simulink model "Modello1DoF_alessio"  (R2023a)
settings: Solver=ode1  StartTime=0.0  StopTime=20  FixedStep=0.001  RelTol=1e-3
libraries: autolibshared x1
settings Model: Creator=salvo  LastModifiedBy=alessio

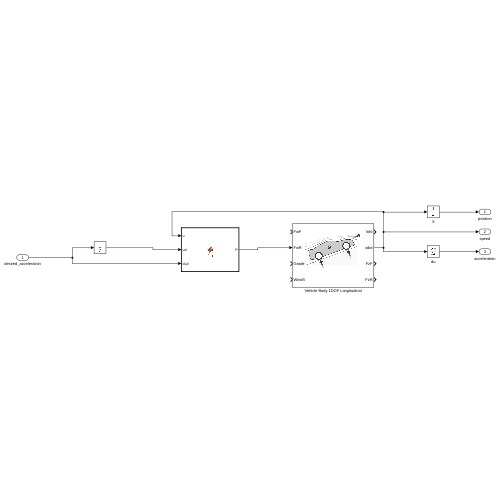
[thumbnail: Simulink's stored preview of the top-level diagram]
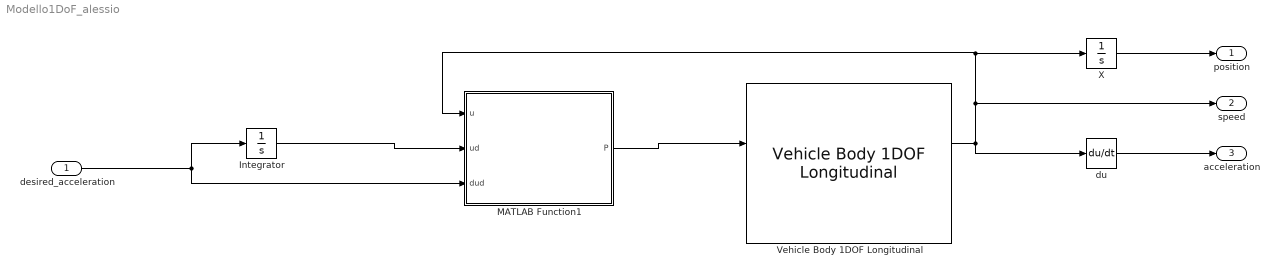
== system Modello1DoF_alessio ==
  desired_acceleration : Inport
  Integrator : Integrator
  MATLAB Function1 : MATLAB Function  TreatAsAtomicUnit=on
  Vehicle Body 1DOF Longitudinal : autolibshared/Vehicle Body 1DOF Longitudinal  VariantControl=SL  extFMode=off  extMMode=off  extTamb=off  wind3D=off  aMode=2  NF=2  NR=2  m=1500  a=1.4  b=1.8  h=.35  Cd=.3  Cl=0  Cpm=0  Af=4  x_o=0  xdot_o=0  Pabs=101325  T=273  g=9.81
      settings: LibrarySourceBlock=vehdynlibeom/Vehicle Body 1DOF Longitudinal
  X : Integrator
  du : Derivative
  position : Outport
  speed : Outport  Port=2
  acceleration : Outport  Port=3
  wires:
  Integrator/1 -> MATLAB Function1/2(ud)
  desired_acceleration/1 -> Integrator/1, MATLAB Function1/3(dud)
  Vehicle Body 1DOF Longitudinal/2 -> MATLAB Function1/1(u), X/1, speed/1, du/1
  MATLAB Function1/1(P) -> Vehicle Body 1DOF Longitudinal/2
  X/1 -> position/1
  du/1 -> acceleration/1

== matlab function Modello1DoF_alessio/MATLAB Function1 ==
  data: u input; P output; ud input; dud input
function P = fcn(u, ud, dud)

ku = 25;
eu = u-ud;
m = 1500;

P = m*(-ku*eu+dud);
